simulink model "IMPLICIT_1ODE_EX1_sim"  (Simulink 8.0)
settings: Solver=ode15s  StartTime=1e-3  StopTime=6*pi  RelTol=1e-3
settings Model: Creator=David  LastModifiedBy=David
settings DataIOCC: SignalLoggingSaveFormat=ModelDataLogs
settings DebuggingCC: FcnCallInpInsideContextMsg=UseLocalSettings  StrictBusMsg=Warning
settings GRTTargetCC: CombineOutputUpdateFcns=off  GRTInterface=on

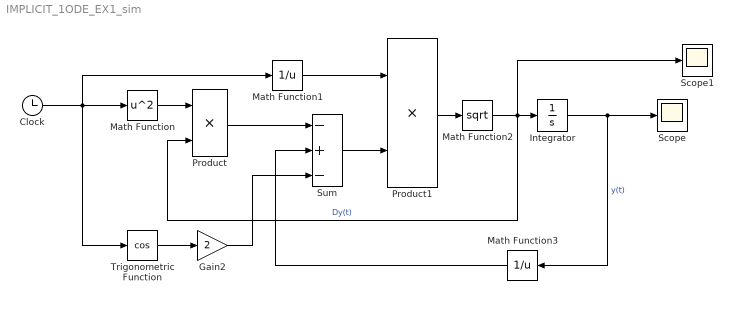
== system IMPLICIT_1ODE_EX1_sim ==
  Clock : Clock
  Gain2 : Gain  Gain=2
  Integrator : Integrator  InitialCondition=1/2
  Math Function : Math  Operator=square  SaturateOnIntegerOverflow=on
  Math Function1 : Math  Operator=reciprocal  SaturateOnIntegerOverflow=on
  Math Function2 : Math  Operator=sqrt  SaturateOnIntegerOverflow=on
  Math Function3 : Math  Operator=reciprocal  SaturateOnIntegerOverflow=on
  Product : Product  RndMeth=Zero
  Product1 : Product  RndMeth=Zero
  Scope : Scope
      settings: SaveName=ODEsols_SIM
  Scope1 : Scope
      settings: SaveName=ODEsols_SIM1
  Sum : Sum  Inputs=-+-
  Trigonometric Function : Trigonometry  Operator=cos
  wires:
  Clock/1 -> Math Function/1, Trigonometric Function/1, Math Function1/1
  Math Function/1 -> Product/1
  Integrator/1 -> Scope/1, Math Function3/1  "y(t)"
  Math Function3/1 -> Sum/2
  Product/1 -> Sum/1
  Math Function1/1 -> Product1/1
  Sum/1 -> Product1/2
  Product1/1 -> Math Function2/1
  Math Function2/1 -> Integrator/1, Product/2, Scope1/1  "Dy(t)"
  Trigonometric Function/1 -> Gain2/1
  Gain2/1 -> Sum/3
